simulink model "model_ROV_backstepping"  (R2022b)
settings: Solver=VariableStepAuto  StartTime=0.0  StopTime=150  RelTol=1e-3
libraries: sim3dlib x1, uavsim3dlib x1
settings Model: Creator=anton  LastModifiedBy=anton

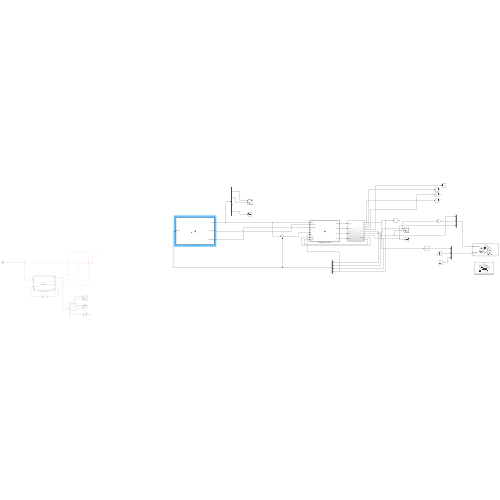
[thumbnail: Simulink's stored preview of the top-level diagram]
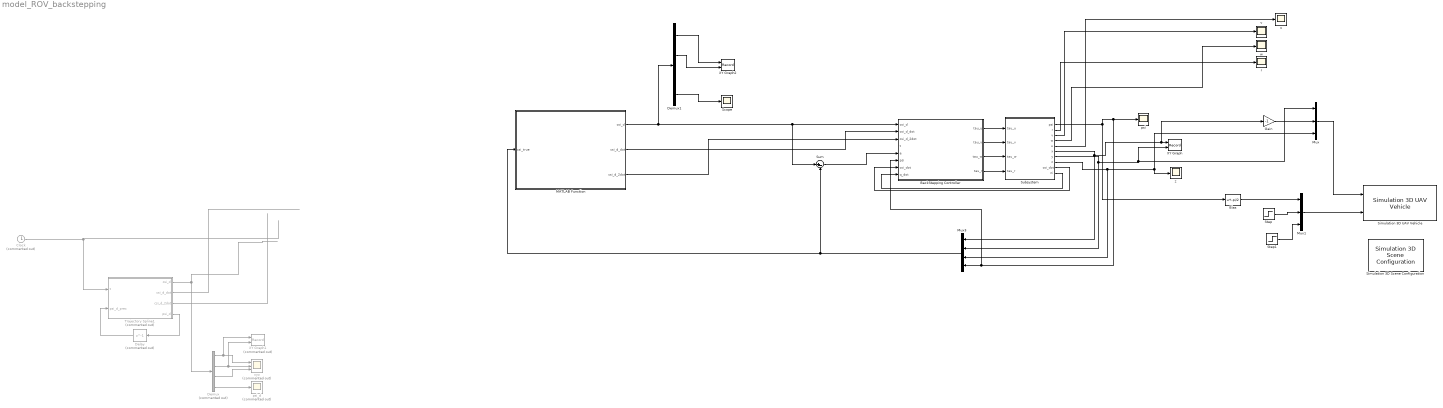
== system model_ROV_backstepping ==
  BackStepping Controller : MATLAB Function  TreatAsAtomicUnit=on
  Bias : Bias  Bias=-pi/2  SaturateOnIntegerOverflow=off
  Clock : Clock  Commented=on
  Delay : Delay  Commented=on  DelayLength=1  InitialCondition=0
  Demux : Demux  Commented=on
  Demux1 : Demux
  Gain : Gain  Gain=-1
  MATLAB Function : MATLAB Function  TreatAsAtomicUnit=on
  Mux : Mux  Inputs=3
  Mux1 : Mux  Inputs=3
  Mux3 : Mux
  Scope : Scope
  Simulation 3D Scene Configuration : sim3dlib/Simulation 3D Scene Configuration  Priority=0  ProjectFormat=Default Scenes  SceneDesc=Airport  ProjectName=C:\Program Files\MATLAB\R2022b\toolbox\shared\sim3d_projects\automotive_project\UE4\WindowsNoEditor\VehicleSimulation.exe  ScenePath=/Game/Maps/HwStrght  EnableOpenDRIVE=off  vehTagList={'Scene Origin';'SimulinkVehicle2'}  vehTag=SimulinkVehicle2  OpVisEn=off  Ts=.02  EnableWindow=on  EnableRemoteAccess=off  EnableWeather=off  SunAltitude=40.0  SunAzimuth=90  clouds=10  wind=1  fog=0  rain=0  EnableGeospatial=off  OriginHeight=200  OriginLatitude=40.744652  OriginLongitude=-73.988864  MapStyle=Aerial  AdditionalAssetIDs=[]  UseAdvancedSunSky=off  SolarTime=11  TimeZone=-5  Day=21  Month=9  Year=2022  UseDaylightSavingTime=on  DSTStartDay=10  DSTStartMonth=3  DSTEndDay=3  DSTEndMonth=11  DSTSwitchHour=2  sensorTag=MainCamera1  sensorId=1  sensorName=MainCamera1  mountLoc=Origin  offsetFlag=off  tmountOffset=[0, 0, 0]  rmountOffset=[0, 0, 0]  HorizontalResolution=1280  VerticalResolution=720  HorizontalFOV=60  mountPoint=[0 0 0]  mountOrientation=[0 0 0]  aMode=0  ID=1  GeoTrigger=Inactive
      settings: LibrarySourceBlock=aerolibsim3d/Simulation 3D Scene Configuration
  Simulation 3D UAV Vehicle : uavsim3dlib/Simulation 3D UAV Vehicle  Priority=-1  Mesh=Quadrotor  MeshPath=/MathWorksUAVContent/UAVs/HexaRotorUAV/HexaRotor.HexaRotor  Color=Yellow  ActorName=SimulinkVehicle2  InitialTranslation=[0 0 0]  InitialRotation=[0 0 0]  SampleTime=-1  ActorType=SimulinkVehicle  ID=2  aMode=4  ActorTag=SimulinkVehicle2
  Step : Step  After=0  SampleTime=0
  Step1 : Step  After=0  SampleTime=0
  Subsystem : Subsystem
  Sum : Sum  Inputs=|+-
  Trajectory Spline1 : MATLAB Function  Commented=on  TreatAsAtomicUnit=on
  XY Graph : Record  FileSettingsInternal="{\"entries\":[{\"content\":{\"excelSettings\":{\"content\":{},\"type\":\"Streamout.ExcelSettings\"}},\"type\":\"Streamout.FileSettingStorage\",\"uuid\":\"\"}],\"packageUris\":[\"http:\\/\\/schema.mathworks.com\\/mf0\\/streamout_blocks\\/R2020a\"],\"version\":\"1.0\"}"  Layout=[1 1]  SignalsInternal="{\"entries\":[{\"content\":{\"signals\":[{\"content\":{\"blockPath\":[],\"channel\":[],\"dimensions\":[1,1],\"domain\":\"\",\"lineColor\":\"#a2142f\",\"plots\":[1],\"port\":1,\"sid\":[],\"signalID\":9378,\"signalName\":\"Subsystem:6\"},\"type\":\"RecordBlkView.Signal\",\"uuid\":\"\"},{\"content\":{\"blockPath\":[],\"channel\":[],\"dimensions\":[1,1],\"domain\":\"\",\"lineColor\":\"#139fff\",\"plots\":[1],\"port\":2,\"sid\":[],\"signalID\":9381,\"signalName\":\"Subsystem:7\"},\"type\":\"RecordBlkView.Signal\",\"uuid\":\"\"}]},\"type\":\"RecordBlkView.InputSignals\",\"uuid\":\"\"}],\"packageUris\":[\"http:\\/\\/schema.mathworks.com\\/mf0\\/streamout_blocks\\/R2020a\"],\"version\":\"1.0\"}"  VisualizationBindings="{\"xyplotplugin\":{\"info\":[{\"series\":[{\"bindingParametersList\":[{\"parameter\":\"X-Axis\",\"signalID\":9378,\"signalName\":\"Subsystem:6\"},{\"parameter\":\"Y-Axis\",\"signalID\":9381,\"signalName\":\"Subsystem:7\"}],\"seriesID\":26505}],\"subplotID\":1}]}}"  CompatibilityTag=XY
  XY Graph1 : Record  Commented=on  FileSettingsInternal="{\"entries\":[{\"content\":{\"excelSettings\":{\"content\":{},\"type\":\"Streamout.ExcelSettings\"}},\"type\":\"Streamout.FileSettingStorage\",\"uuid\":\"\"}],\"packageUris\":[\"http:\\/\\/schema.mathworks.com\\/mf0\\/streamout_blocks\\/R2020a\"],\"version\":\"1.0\"}"  Layout=[1 1]  SignalsInternal="{\"entries\":[{\"content\":{\"signals\":[{\"content\":{\"blockPath\":[],\"channel\":[],\"dimensions\":[1,1],\"domain\":\"\",\"lineColor\":\"#a2142f\",\"plots\":[1],\"port\":1,\"sid\":[],\"signalID\":9362,\"signalName\":\"Demux:1\"},\"type\":\"RecordBlkView.Signal\",\"uuid\":\"\"},{\"content\":{\"blockPath\":[],\"channel\":[],\"dimensions\":[1,1],\"domain\":\"\",\"lineColor\":\"#139fff\",\"plots\":[1],\"port\":2,\"sid\":[],\"signalID\":9365,\"signalName\":\"Demux:2\"},\"type\":\"RecordBlkView.Signal\",\"uuid\":\"\"}]},\"type\":\"RecordBlkView.InputSignals\",\"uuid\":\"\"}],\"packageUris\":[\"http:\\/\\/schema.mathworks.com\\/mf0\\/streamout_blocks\\/R2020a\"],\"version\":\"1.0\"}"  VisualizationBindings="{\"xyplotplugin\":{\"info\":[{\"series\":[{\"bindingParametersList\":[{\"parameter\":\"X-Axis\",\"signalID\":9362,\"signalName\":\"Demux:1\"},{\"parameter\":\"Y-Axis\",\"signalID\":9365,\"signalName\":\"Demux:2\"}],\"seriesID\":48808}],\"subplotID\":1}]}}"  CompatibilityTag=XY
  XY Graph2 : Record  FileSettingsInternal="{\"entries\":[{\"content\":{\"excelSettings\":{\"content\":{},\"type\":\"Streamout.ExcelSettings\"}},\"type\":\"Streamout.FileSettingStorage\",\"uuid\":\"\"}],\"packageUris\":[\"http:\\/\\/schema.mathworks.com\\/mf0\\/streamout_blocks\\/R2020a\"],\"version\":\"1.0\"}"  Layout=[1 1]  SignalsInternal="{\"entries\":[{\"content\":{\"signals\":[{\"content\":{\"blockPath\":[],\"channel\":[],\"dimensions\":[1,1],\"domain\":\"\",\"lineColor\":\"#a2142f\",\"plots\":[1],\"port\":1,\"sid\":[],\"signalID\":9370,\"signalName\":\"Demux1:1\"},\"type\":\"RecordBlkView.Signal\",\"uuid\":\"\"},{\"content\":{\"blockPath\":[],\"channel\":[],\"dimensions\":[1,1],\"domain\":\"\",\"lineColor\":\"#139fff\",\"plots\":[1],\"port\":2,\"sid\":[],\"signalID\":9373,\"signalName\":\"Demux1:2\"},\"type\":\"RecordBlkView.Signal\",\"uuid\":\"\"}]},\"type\":\"RecordBlkView.InputSignals\",\"uuid\":\"\"}],\"packageUris\":[\"http:\\/\\/schema.mathworks.com\\/mf0\\/streamout_blocks\\/R2020a\"],\"version\":\"1.0\"}"  VisualizationBindings="{\"xyplotplugin\":{\"info\":[{\"series\":[{\"bindingParametersList\":[{\"parameter\":\"X-Axis\",\"signalID\":9370,\"signalName\":\"Demux1:1\"},{\"parameter\":\"Y-Axis\",\"signalID\":9373,\"signalName\":\"Demux1:2\"}],\"seriesID\":53717}],\"subplotID\":1}]}}"  CompatibilityTag=XY
  psi : Scope
  psi_d : Scope  Commented=on
  r : Scope
  u : Scope
  v : Scope
  w : Scope
  xyz : Scope  Commented=on  NumInputPorts=3
  z : Scope
  wires:
  Subsystem/1(psi) -> psi/1, BackStepping Controller/6(psi), Mux3/4, Bias/1
  Subsystem/2(r) -> r/1
  Subsystem/3(v) -> v/1
  Subsystem/4(w) -> w/1
  Subsystem/5(u) -> u/1
  Subsystem/6(x) -> Mux3/1, Gain/1, XY Graph/1
  Subsystem/8(z) -> Mux3/3, Mux/3, z/1
  Mux/1 -> Simulation 3D UAV Vehicle/1
  Mux1/1 -> Simulation 3D UAV Vehicle/2
  Step/1 -> Mux1/2
  Step1/1 -> Mux1/3
  Clock/1 -> Trajectory Spline1/1(t)
  BackStepping Controller/1(tau_u) -> Subsystem/1(tau_u)
  BackStepping Controller/2(tau_v) -> Subsystem/2(tau_v)
  BackStepping Controller/3(tau_w) -> Subsystem/3(tau_w)
  BackStepping Controller/4(tau_r) -> Subsystem/4(tau_r)
  Mux3/1 -> MATLAB Function/1(csi_true), Sum/2
  Sum/1 -> BackStepping Controller/5(e)
  Subsystem/9(csi_dot) -> BackStepping Controller/7(csi_dot)
  Subsystem/10(ni) -> BackStepping Controller/8(q_dot)
  Trajectory Spline1/1(csi_d) -> Demux/1
  Trajectory Spline1/2(csi_d_dot) -> ?
  Trajectory Spline1/3(csi_d_2dot) -> ?
  Demux/1 -> XY Graph1/1, xyz/1
  Demux/2 -> XY Graph1/2, xyz/2
  Demux/3 -> xyz/3
  Demux/4 -> psi_d/1
  Subsystem/7(y) -> Mux3/2, Mux/1, XY Graph/2
  Gain/1 -> Mux/2
  Bias/1 -> Mux1/1
  Trajectory Spline1/4(psi_d) -> Delay/1
  Delay/1 -> Trajectory Spline1/2(psi_d_prec)
  MATLAB Function/1(csi_d) -> Demux1/1, Sum/1, BackStepping Controller/1(csi_d)
  MATLAB Function/2(csi_d_dot) -> BackStepping Controller/2(csi_d_dot)
  MATLAB Function/3(csi_d_2dot) -> BackStepping Controller/3(csi_d_2dot)
  Demux1/1 -> XY Graph2/1
  Demux1/2 -> XY Graph2/2
  Demux1/4 -> Scope/1

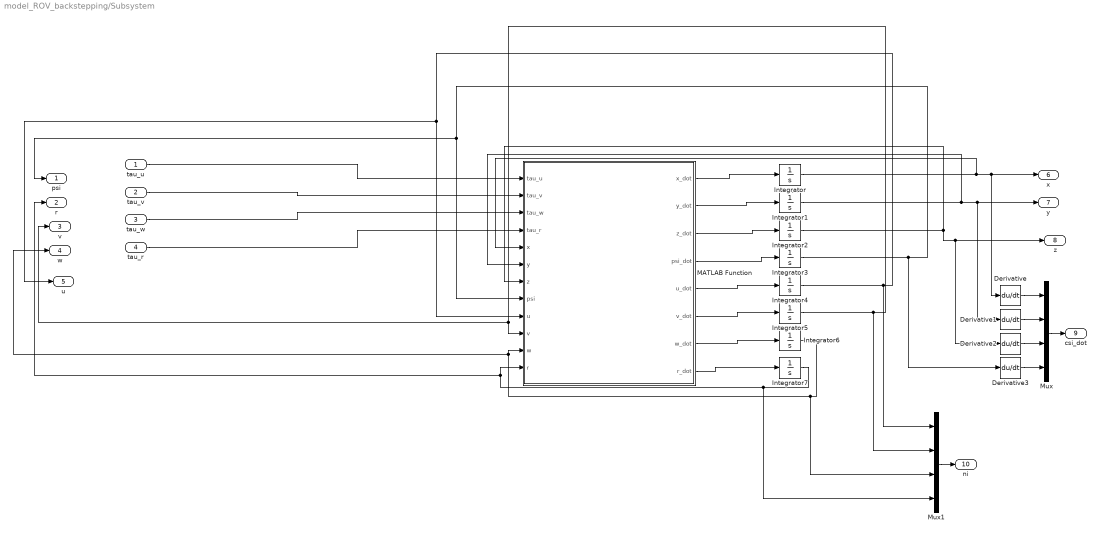
== system model_ROV_backstepping/Subsystem ==
  tau_u : Inport
  tau_v : Inport  Port=2
  tau_w : Inport  Port=3
  tau_r : Inport  Port=4
  Derivative{,1..3} (4 alike) : Derivative  CoefficientInTFapproximation=0.01
  Integrator{,1..7} (8 alike) : Integrator
  MATLAB Function : MATLAB Function  TreatAsAtomicUnit=on
  Mux : Mux
  Mux1 : Mux
  psi : Outport
  r : Outport  Port=2
  v : Outport  Port=3
  w : Outport  Port=4
  u : Outport  Port=5
  x : Outport  Port=6
  y : Outport  Port=7
  z : Outport  Port=8
  csi_dot : Outport  Port=9
  ni : Outport  Port=10
  wires:
  MATLAB Function/1(x_dot) -> Integrator/1
  Integrator3/1 -> Derivative3/1, psi/1, MATLAB Function/8(psi)
  MATLAB Function/6(v_dot) -> Integrator5/1
  MATLAB Function/4(psi_dot) -> Integrator3/1
  Integrator2/1 -> MATLAB Function/7(z), Derivative2/1, z/1
  Integrator6/1 -> Mux1/3, w/1, MATLAB Function/11(w)
  MATLAB Function/5(u_dot) -> Integrator4/1
  MATLAB Function/7(w_dot) -> Integrator6/1
  tau_v/1 -> MATLAB Function/2(tau_v)
  MATLAB Function/8(r_dot) -> Integrator7/1
  tau_w/1 -> MATLAB Function/3(tau_w)
  MATLAB Function/3(z_dot) -> Integrator2/1
  Integrator1/1 -> Derivative1/1, y/1, MATLAB Function/6(y)
  Integrator5/1 -> Mux1/2, v/1, MATLAB Function/10(v)
  tau_r/1 -> MATLAB Function/4(tau_r)
  Integrator/1 -> Derivative/1, x/1, MATLAB Function/5(x)
  MATLAB Function/2(y_dot) -> Integrator1/1
  tau_u/1 -> MATLAB Function/1(tau_u)
  Mux/1 -> csi_dot/1
  Mux1/1 -> ni/1
  Integrator4/1 -> Mux1/1, u/1, MATLAB Function/9(u)
  Integrator7/1 -> Mux1/4, r/1, MATLAB Function/12(r)
  Derivative/1 -> Mux/1
  Derivative1/1 -> Mux/2
  Derivative2/1 -> Mux/3
  Derivative3/1 -> Mux/4

== matlab function model_ROV_backstepping/BackStepping Controller ==
  data: csi_d input size=[4 1]; csi_d_dot input; csi_d_2dot input; tau_u output; tau_v output; tau_w output; tau_r output; t input; e input size=[4 1]; psi input; csi_dot input size=[4 1]; q_dot input size=[4 1]
function [tau_u,tau_v,tau_w,tau_r] = backstepping(csi_d, csi_d_dot,csi_d_2dot,t,e,psi,csi_dot,q_dot)

J = [cos(psi) -sin(psi) 0 0;
     sin(psi) cos(psi) 0 0;
     0 0 1 0;
     0 0 0 1];
psi_d = csi_d(4);
x_d_dot = csi_d_dot(1);
y_d_dot = csi_d_dot(2);
z_d_dot = csi_d_dot(3);
psi_d_dot = csi_d_dot(4);

x_d_2dot = csi_d_2dot(1);
y_d_2dot = csi_d_2dot(2);
z_d_2dot = csi_d_2dot(3);
psi_2d_dot = csi_d_2dot(4);
LAMBDA = diag([1 1 1 1]);

q_r_dot = inv(J) * (csi_d_dot + LAMBDA * e);
J_inv_dot = [-sin(psi)*csi_dot(4) cos(psi)*csi_dot(4) 0 0;
            -cos(psi)*csi_dot(4) -sin(psi)*csi_dot(4) 0 0;
             0 0 0 0;
             0 0 0 0];


e_dot = csi_d_dot - csi_dot;
q_r_2dot = J_inv_dot * (csi_d_dot + LAMBDA * e) + inv(J) * (csi_d_2dot + LAMBDA * e_dot);
s = inv(J) * (e_dot + LAMBDA*e);

u = q_dot(1);
v = q_dot(2);
w = q_dot(3);
r = q_dot(4);
m = 12;
d = 0.338;
l = 0.457;

I = 1/12*m*(d^2+l^2);

Y_v_dot = 0;
Y_r = 0;
X_u_dot = 0;
X_u = 0;
Y_v = 0;
Z_w = 0;
N_r = 0;
N_r_r = 0;

M = diag([m m m I]);
C = [0 0 0 Y_v_dot*v + Y_r*r;
     0 0 0 -X_u_dot*u;
     0 0 0 0;
     -Y_v_dot*v-Y_r*r X_u_dot*u 0 0];
D = diag([-X_u -Y_v -Z_w -N_r-N_r_r*r]);

K_d = eye(4);

tau = M * q_r_2dot + C * q_r_dot + K_d * s + J'*e;

tau_u = tau(1);
tau_v = tau(2);
tau_w = tau(3);
tau_r = tau(4);

end

== matlab function model_ROV_backstepping/Subsystem/MATLAB Function ==
  data: tau_u input; tau_v input; tau_w input; tau_r input; x input; y input; z input; psi input; u input; x_dot output; v input; w input; r input; y_dot output; z_dot output; psi_dot output; u_dot output; v_dot output; w_dot output; r_dot output
function [x_dot,y_dot,z_dot,psi_dot,u_dot,v_dot,w_dot,r_dot] = Dynamics(tau_u,tau_v,tau_w,tau_r,x,y,z,psi,u,v,w,r)

m = 12;
d = 0.338;
l = 0.457;

I = 1/12*m*(d^2+l^2);

Y_v_dot = 0;
Y_r = 0;
X_u_dot = 0;
X_u = 0;
Y_v = 0;
Z_w = 0;
N_r = 0;
N_r_r = 0;


M = diag([m m m I]);
C = [0 0 0 Y_v_dot*v + Y_r*r;
     0 0 0 -X_u_dot*u;
     0 0 0 0;
     -Y_v_dot*v-Y_r*r X_u_dot*u 0 0];
D = diag([-X_u -Y_v -Z_w -N_r-N_r_r*r]);

ni = [u,v,w,r]';
tau = [tau_u,tau_v,tau_w,tau_r]';


ni_dot = inv(M)*(-C*ni - D*ni + tau);

eta_dot = [cos(psi) -sin(psi) 0 0;
           sin(psi) cos(psi) 0 0;
           0 0 1 0;
           0 0 0 1]*ni;

x_dot = eta_dot(1);
y_dot = eta_dot(2);
z_dot = eta_dot(3);
psi_dot = eta_dot(4);

u_dot = ni_dot(1);
v_dot = ni_dot(2);
w_dot = ni_dot(3);
r_dot = ni_dot(4);

== matlab function model_ROV_backstepping/MATLAB Function ==
  data: csi_d output size=[4,1]; csi_d_dot output size=[4,1]; csi_d_2dot output size=[4,1]; csi_true input size=[4,1]
function [csi_d, csi_d_dot, csi_d_2dot] = TrajectoryTest(csi_true)
    t_fin = 50;
    x = [];
    y = [];
    z = [];
    x_true = csi_true(1);
    y_true = csi_true(2);
    z_true = csi_true(3);
    psi = [];
    for t=0:t_fin/1000:t_fin
        x = [x,5*cos(t)-5];
        y = [y,5*sin(t)];
        z = [z,0];
        psi = [psi,atan2(5*cos(t),-5*sin(t))];
    end
    
    e = vecnorm([x_true;y_true;z_true]*ones(1,1001) - [x;y;z]);

    [~,i] = min(e);

    csi_d = [x(i),y(i),z(i),psi(i)]';
    
    csi_d_dot = [cos(psi(i)) -sin(psi(i)) 0 0;
                   sin(psi(i)) cos(psi(i)) 0 0;
                   0 0 1 0;
                   0 0 0 1]*[0.5;0;0;0];

    csi_d_2dot = [0,0,0,0]';
end

== matlab function model_ROV_backstepping/Trajectory Spline1 ==
  data: t input; csi_d output; csi_d_dot output; csi_d_2dot output; psi_d_prec input; psi_d output
function [csi_d,csi_d_dot,csi_d_2dot,psi_d] = trajectory(t,psi_d_prec)

% Punti di Interpolazione
x1 = 0;
y1 = 0;
z1 = 0;
x2 = 10;
y2 = 10;
z2 = 10;
x3 = 20;
y3 = 0;
z3 = 20;
J_eval = [];

% MINIMIZZAZIONE DEL COSTO

i=[0.1:0.1:100];
for h = i
    J = 2*h + (3*(x1^2 - 4*x1*x2 + 2*x1*x3 + 4*x2^2 - 4*x2*x3 + x3^2 + y1^2 - ...
    4*y1*y2 + 2*y1*y3 + 4*y2^2 - 4*y2*y3 + y3^2 + z1^2 - 4*z1*z2 + 2*z1*z3 + ...
    4*z2^2 - 4*z2*z3 + z3^2))/(2*h^3) + (11*x1^2 - 24*x1*x2 + 2*x1*x3 + ...
    24*x2^2 - 24*x2*x3 + 11*x3^2 + 11*y1^2 - 24*y1*y2 + 2*y1*y3 + 24*y2^2 - ...
    24*y2*y3 + 11*y3^2 + 11*z1^2 - 24*z1*z2 + 2*z1*z3 + 24*z2^2 - 24*z2*z3 + ...
    11*z3^2)/(10*h) + (13*x1^2 - 36*x1*x2 + 10*x1*x3 + 36*x2^2 - 36*x2*x3 + ...
    13*x3^2 + 13*y1^2 - 36*y1*y2 + 10*y1*y3 + 36*y2^2 - 36*y2*y3 + 13*y3^2 + ...
    13*z1^2 - 36*z1*z2 + 10*z1*z3 + 36*z2^2 - 36*z2*z3 + 13*z3^2)/(8*h^2);
    J_eval = [J_eval,J];
end
[J_min,i_min] = (min(J_eval));
h_ottimo = (i(i_min))

% Spline sulla x
Mx = 3/(2*h_ottimo^2)*(x1+x3-2*x2);

bx1 = 0;
bx2 = Mx/2;
dx1 = x1;
dx2 = x2;
ax1 = Mx/(6*h_ottimo);
ax2 = -Mx/(6*h_ottimo);
cx1 = (x2-x1)/h_ottimo - Mx*h_ottimo/6;
cx2 = (x3-x2)/h_ottimo - Mx*h_ottimo/3;

% Spline sulla y
My = 3/(2*h_ottimo^2)*(y1+y3-2*y2);

by1 = 0;
by2 = My/2;
dy1 = y1;
dy2 = y2;
ay1 = My/(6*h_ottimo);
ay2 = -My/(6*h_ottimo);
cy1 = (y2-y1)/h_ottimo - My*h_ottimo/6;
cy2 = (y3-y2)/h_ottimo - My*h_ottimo/3;

% Spline sulla z
Mz = 3/(2*h_ottimo^2)*(z1+z3-2*z2);

bz1 = 0;
bz2 = Mz/2;
dz1 = z1;
dz2 = z2;
az1 = Mz/(6*h_ottimo);
az2 = -Mz/(6*h_ottimo);
cz1 = (z2-z1)/h_ottimo - Mz*h_ottimo/6;
cz2 = (z3-z2)/h_ottimo - Mz*h_ottimo/3;

t0 = 0;
if t < t0 + h_ottimo
    p_x = ax1*(t-t0)^3 + bx1*(t-t0)^2 + cx1*(t-t0) + dx1;
    p_y = ay1*(t-t0)^3 + by1*(t-t0)^2 + cy1*(t-t0) + dy1;
    p_z = az1*(t-t0)^3 + bz1*(t-t0)^2 + cz1*(t-t0) + dz1;
    v_x = 3*ax1*(t-t0)^2 + 2*bx1*(t-t0) + cx1;
    v_y = 3*ay1*(t-t0)^2 + 2*by1*(t-t0) + cy1;
    v_z = 3*az1*(t-t0)^2 + 2*bz1*(t-t0) + cz1;
    acc_x = 6*ax1*(t-t0) + 2*bx1;
    acc_y = 6*ay1*(t-t0) + 2*by1;
    acc_z = 6*az1*(t-t0) + 2*bz1;
    acc_x_dot = 6*ax1;
    acc_y_dot = 6*ay1;
    acc_z_dot = 6*az1;

elseif (t >= t0 + h_ottimo) && (t < t0+2*h_ottimo)
    p_x = ax2*(t-t0-h_ottimo)^3 + bx2*(t-t0-h_ottimo)^2 + cx2*(t-t0-h_ottimo) + dx2;
    p_y = ay2*(t-t0-h_ottimo)^3 + by2*(t-t0-h_ottimo)^2 + cy2*(t-t0-h_ottimo) + dy2;
    p_z = az2*(t-t0-h_ottimo)^3 + bz2*(t-t0-h_ottimo)^2 + cz2*(t-t0-h_ottimo) + dz2;
    v_x = 3*ax2*(t-t0-h_ottimo)^2 + 2*bx2*(t-t0-h_ottimo) + cx2;
    v_y = 3*ay2*(t-t0-h_ottimo)^2 + 2*by2*(t-t0-h_ottimo) + cy2;
    v_z = 3*az2*(t-t0-h_ottimo)^2 + 2*bz2*(t-t0-h_ottimo) + cz2;
    acc_x = 6*ax2*(t-t0-h_ottimo) + 2*bx2;
    acc_y = 6*ay2*(t-t0-h_ottimo) + 2*by2;
    acc_z = 6*az2*(t-t0-h_ottimo) + 2*bz2;
    acc_x_dot = 6*ax2;
    acc_y_dot = 6*ay2;
    acc_z_dot = 6*az2;
else
    p_x = x3;
    p_y = y3;
    p_z = z3;
    v_x = 0;
    v_y = 0;
    v_z = 0;
    acc_x = 0;
    acc_y = 0;
    acc_z = 0;
    acc_x_dot = 0;
    acc_y_dot = 0;
    acc_z_dot = 0;
end


if t < t0+2*h_ottimo
    psi_d = atan2(v_y,v_x);
    psi_d_dot = (acc_y*v_x - v_y*acc_x)/(v_x^2 + v_y^2);
    psi_d_2dot = ((acc_y_dot*v_x - v_y*acc_x_dot)*(v_x^2+v_y^2)- ...
        (acc_y*v_x - v_y*acc_x)*(2*v_x*acc_x + 2*v_y*acc_y))/(v_x^4 + ...
        v_y^4 + 2*v_x^2*v_y^2);
else
    psi_d = psi_d_prec;
    psi_d_dot = 0;
    psi_d_2dot = 0;
end
csi_d = [p_x p_y p_z psi_d]';
csi_d_dot = [v_x v_y v_z psi_d_dot]';
csi_d_2dot = [acc_x acc_y acc_z psi_d_2dot]';
